simulink model "sistema_mecanico_translacional"  (R2020a)
settings: Solver=VariableStepAuto  StartTime=0.0  StopTime=150  RelTol=1e-3
libraries: fl_lib x12, nesl_utility x4, sdl_lib x1
settings Model: Creator=ed385  LastModifiedBy=Win10

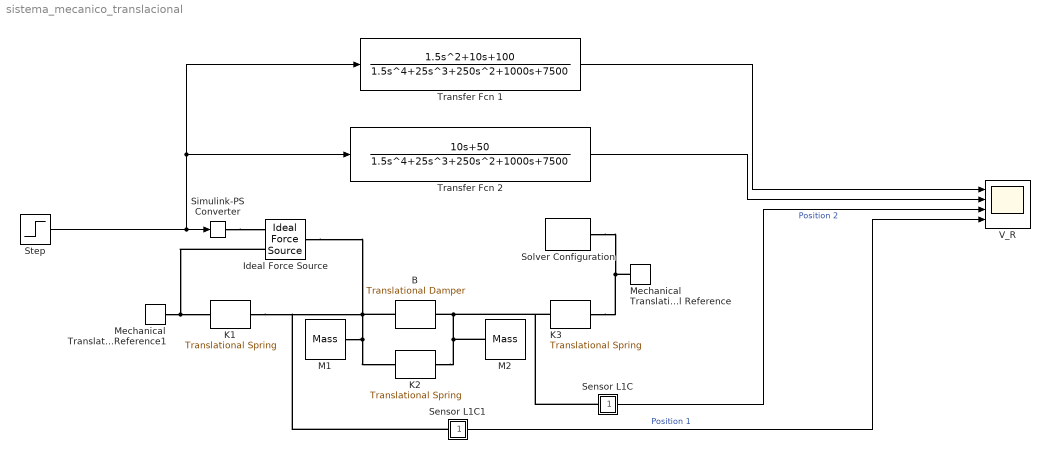
== system sistema_mecanico_translacional ==
  B : sdl_lib/Couplings & Drives/Springs & Dampers/Translational Damper  D=10 N/(m/s)  enable_faults=0  b_fault=1e6 N/(m/s)  temporal_fault=0  fault_time=5 s  shock_fault=0  acceleration_limit=100 m/s^2  shock_limit=1  report_fault=1
      settings: SourceProductBaseCode=LD
  Ideal Force Source : fl_lib/Mechanical/Mechanical Sources/Ideal Force Source
  K1 : fl_lib/Mechanical/Translational Elements/Translational Spring  spr_rate=50 N/m  v_specify=off  v_priority=None  v=0 m/s  v_nominal_specify=off  v_nominal_unit=m/s  v_nominal_value=1  f_specify=off  f_priority=None  f=0 N  f_nominal_specify=off  f_nominal_unit=N  f_nominal_value=1  x_specify=off  x_priority=High  x=0 m  x_nominal_specify=off  x_nominal_unit=m  x_nominal_value=1
  K2 : fl_lib/Mechanical/Translational Elements/Translational Spring  spr_rate=50 N/m  v_specify=off  v_priority=None  v=0 m/s  v_nominal_specify=off  v_nominal_unit=m/s  v_nominal_value=1  f_specify=off  f_priority=None  f=0 N  f_nominal_specify=off  f_nominal_unit=N  f_nominal_value=1  x_specify=off  x_priority=High  x=0 m  x_nominal_specify=off  x_nominal_unit=m  x_nominal_value=1
  K3 : fl_lib/Mechanical/Translational Elements/Translational Spring  spr_rate=50 N/m  v_specify=off  v_priority=None  v=0 m/s  v_nominal_specify=off  v_nominal_unit=m/s  v_nominal_value=1  f_specify=off  f_priority=None  f=0 N  f_nominal_specify=off  f_nominal_unit=N  f_nominal_value=1  x_specify=off  x_priority=High  x=0 m  x_nominal_specify=off  x_nominal_unit=m  x_nominal_value=1
  M1 : fl_lib/Mechanical/Translational Elements/Mass  mass=1 kg  v_specify=off  v_priority=High  v=0 m/s  v_nominal_specify=off  v_nominal_unit=m/s  v_nominal_value=1  f_specify=off  f_priority=High  f=0 N  f_nominal_specify=off  f_nominal_unit=N  f_nominal_value=1
  M2 : fl_lib/Mechanical/Translational Elements/Mass  mass=1.5 kg  v_specify=off  v_priority=High  v=0 m/s  v_nominal_specify=off  v_nominal_unit=m/s  v_nominal_value=1  f_specify=off  f_priority=None  f=0 N  f_nominal_specify=off  f_nominal_unit=N  f_nominal_value=1
  Mechanical Translational Reference : fl_lib/Mechanical/Translational Elements/Mechanical Translational Reference
  Mechanical Translational Reference1 : fl_lib/Mechanical/Translational Elements/Mechanical Translational Reference
  Sensor L1C : Subsystem
      mask Display: disp('P')
  Sensor L1C1 : Subsystem
      mask Display: disp('P')
  Simulink-PS Converter : nesl_utility/Simulink-PS Converter  PhysicalDomain=network_engine_domain  SubClassName=ps_input  LeftPortType=input  RightPortType=output  PseudoPeriodic=off  Frequencies=[]  NoiseDistribution=none  NoiseParameters=[]  Unit=1  AffineConversion=off  FilteringAndDerivatives=provide  SimscapeFilterOrder=1  InputFilterTimeConstant=0.001  UdotUserProvided=0
  Solver Configuration : nesl_utility/Solver Configuration  PhysicalDomain=network_engine_domain  SubClassName=solver  LeftPortType=input  RightPortType=generic  Tones=[]  Harmonics=[]  SimulateNoise=off  Profile=off  UseLocalSampling=off  EnableSwitchedLinearOptims=on  FrequencyDomain=off  UseCCode=off  RelTol=0.001  AbsTol=1e-06  MinStep=1e-09  ToWorkspace=off  RevertToSquareIcSolve=off  NumHomotopyIterations=100  PhasorMode=off  PhasorModeNumHarmonics=1  DoDC=off  ResidualTolerance=1e-09  UseLocalSolver=off  LocalSolverChoice=NE_BACKWARD_EULER_ADVANCER  LocalSolverSampleTime=0.001  DoFixedCost=off  MaxNonlinIter=3  MaxModeIter=2  LinearAlgebra=auto  EquationFormulation=NE_TIME_EF  DelaysMemoryBudget=1024  AutomaticFiltering=on  FilteringTimeConstant=0.001  PartitionStorageMethod=AS_NEEDED  PartitionMemoryBudget=1024  PartitionMethod=ROBUST
  Step : Step  Time=0.001  Before=1  After=0  SampleTime=0
  Transfer Fcn 1 : TransferFcn  Numerator=[1.5 10 100]  Denominator=[1.5 25 250 1000 7500]
  Transfer Fcn 2 : TransferFcn  Numerator=[10 50 ]  Denominator=[1.5 25 250 1000 7500]
  V_R : Scope  NumInputPorts=4
  wires:
  Step/1 -> Transfer Fcn 2/1, Transfer Fcn 1/1, Simulink-PS Converter/1
  Sensor L1C1/1(Position) -> V_R/4  "Position 1"
  Transfer Fcn 2/1 -> V_R/2
  Transfer Fcn 1/1 -> V_R/1
  Sensor L1C/1(Position) -> V_R/3  "Position 2"
  connections:
  Mechanical Translational Reference/LConn1 -- Solver Configuration/RConn1 -- K3/RConn1
  K2/RConn1 -- M2/LConn1 -- Sensor L1C/LConn1 -- K3/LConn1 -- B/RConn1
  Mechanical Translational Reference1/LConn1 -- Ideal Force Source/RConn2 -- K1/LConn1
  B/LConn1 -- K1/RConn1 -- Sensor L1C1/LConn1 -- Ideal Force Source/LConn1 -- M1/LConn1 -- K2/LConn1
  Simulink-PS Converter/RConn1 -- Ideal Force Source/RConn1

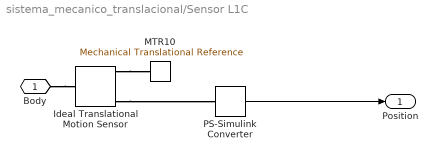
== system sistema_mecanico_translacional/Sensor L1C ==
  Ideal Translational Motion Sensor : fl_lib/Mechanical/Mechanical Sensors/Ideal Translational Motion Sensor  Tag=Factory Generic  offset=0 m
      settings: SourceProductBaseCode=MT,SS
  MTR10 : fl_lib/Mechanical/Translational Elements/Mechanical Translational Reference  Tag=Factory Generic
      settings: SourceProductBaseCode=MT,SS
  PS-Simulink Converter : nesl_utility/PS-Simulink Converter  PhysicalDomain=network_engine_domain  SubClassName=ps_output  LeftPortType=input  RightPortType=output  PseudoPeriodic=off  Frequencies=[]  Unit=1  AffineConversion=off
      settings: SourceProductBaseCode=MT,SS
  Body : PMIOPort  Side=Left
  Position : Outport  VectorParamsAs1DForOutWhenUnconnected=off
  wires:
  PS-Simulink Converter/1 -> Position/1
  connections:
  Ideal Translational Motion Sensor/RConn1 -- MTR10/LConn1
  Ideal Translational Motion Sensor/RConn3 -- PS-Simulink Converter/LConn1
  Body/RConn1 -- Ideal Translational Motion Sensor/LConn1

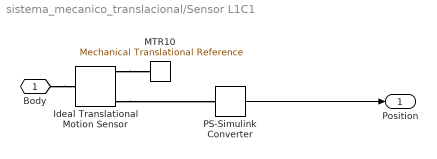
== system sistema_mecanico_translacional/Sensor L1C1 ==
  Ideal Translational Motion Sensor : fl_lib/Mechanical/Mechanical Sensors/Ideal Translational Motion Sensor  Tag=Factory Generic  offset=0 m
      settings: SourceProductBaseCode=MT,SS
  MTR10 : fl_lib/Mechanical/Translational Elements/Mechanical Translational Reference  Tag=Factory Generic
      settings: SourceProductBaseCode=MT,SS
  PS-Simulink Converter : nesl_utility/PS-Simulink Converter  PhysicalDomain=network_engine_domain  SubClassName=ps_output  LeftPortType=input  RightPortType=output  PseudoPeriodic=off  Frequencies=[]  Unit=1  AffineConversion=off
      settings: SourceProductBaseCode=MT,SS
  Body : PMIOPort  Side=Left
  Position : Outport  VectorParamsAs1DForOutWhenUnconnected=off
  wires:
  PS-Simulink Converter/1 -> Position/1
  connections:
  Body/RConn1 -- Ideal Translational Motion Sensor/LConn1
  Ideal Translational Motion Sensor/RConn3 -- PS-Simulink Converter/LConn1
  Ideal Translational Motion Sensor/RConn1 -- MTR10/LConn1
